simulink model "VtP_mod_3Bit"  (Simulink 7.9)
settings: Solver=ode45  StartTime=0.0  StopTime=simu.trantime  RelTol=1e-3
undefined symbols (not defined in the file): dc, Fs, mod, OSR, sinamp, sinfreq
libraries: dspsigattribs x14, dspsigops x9, dspmtrx3 x7, commblksprivate x7, commsrccod2 x7, dsparch4 x1, simulink x1, dspsrcs4 x1
settings Model: Creator=Isacco Arnaldi  LastModifiedBy=Arnaldi Isacco
settings SolverCC: ZcThreshold=1e-3  ZeroCrossAlgorithm=Adaptive  AutoInsertRateTranBlk=on
settings DataIOCC: LimitDataPoints=off  MaxDataPoints=50000  SaveOutput=off  SignalLogging=off  DSMLogging=off  SaveTime=off
settings OptimizationCC: InlineParams=on
settings DebuggingCC: SaveWithDisabledLinksMsg=none  SaveWithParameterizedLinksMsg=none  StrictBusMsg=Warning
settings ModelReferenceCC: ModelReferenceNumInstancesAllowed=Single
settings CodeAppCC: CustomSymbolStrType=$N$R$M_T
settings GRTTargetCC: CombineOutputUpdateFcns=off  GRTInterface=on
settings ConfigurationSet: Description=SimMechanics 2G

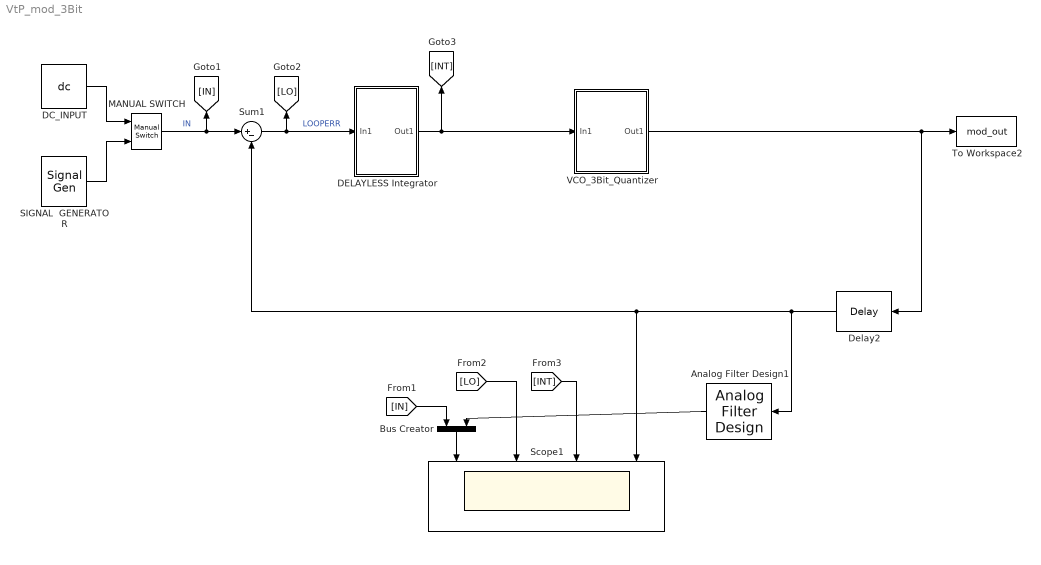
== system VtP_mod_3Bit ==
  Analog Filter Design1 : dsparch4/Analog Filter Design  method=Butterworth  filttype=Lowpass  N=8  Wlo=pi*(Fs/OSR)  Whi=80  Rp=2  Rs=40
  Bus Creator : BusCreator  Inputs=2
  DC_INPUT : Constant  Value=dc  VectorParams1D=off  OutDataTypeStr=double  SampleTime=1/Fs
  DELAYLESS Integrator : Subsystem
  Delay2 : dspsigops/Delay  InputProcessing=Inherited (this choice will be removed - see release notes)  dly_unit=Samples  delay=1  ic_detail=off  dif_ic_for_ch=off  dif_ic_for_dly=off  ic=0  reset_popup=None
  MANUAL SWITCH : simulink/Signal Routing/Manual Switch  sw=0  action=0  varsize=off
      settings: AttributesFormatString=Double click to\nselect the desired\ninput
  SIGNAL  GENERATOR : SignalGenerator  Amplitude=sinamp  Frequency=sinfreq  VectorParams1D=off
  Scope1 : Scope  NumInputPorts=4
      settings: TimeRange=2.089895171320487e-05  YMin=-1.1~-0.6~-0.6~-0.3  YMax=1.1~1.6~1.6~0.1
  Sum1 : Sum  Inputs=|+-  SampleTime=1/Fs
  To Workspace2 : ToWorkspace  VariableName=mod_out  SampleTime=-1
  VCO_3Bit_Quantizer : Subsystem
  wires:
  Sum1/1 -> [LO], DELAYLESS Integrator/1(In1)  "LOOPERR"
  DELAYLESS Integrator/1(Out1) -> [INT], VCO_3Bit_Quantizer/1(In1)
  Delay2/1 -> Analog Filter Design1/1, Sum1/2, Scope1/4
  DC_INPUT/1 -> MANUAL SWITCH/1
  SIGNAL  GENERATOR/1 -> MANUAL SWITCH/2
  MANUAL SWITCH/1 -> Sum1/1, [IN]  "IN"
  [IN] -> Bus Creator/1
  Bus Creator/1 -> Scope1/1
  Analog Filter Design1/1 -> Bus Creator/2
  [LO] -> Scope1/2
  [INT] -> Scope1/3
  VCO_3Bit_Quantizer/1(Out1) -> Delay2/1, To Workspace2/1

== system VtP_mod_3Bit/DELAYLESS Integrator ==
  In1 : Inport
  Delay1 : dspsigops/Delay  InputProcessing=Inherited (this choice will be removed - see release notes)  dly_unit=Samples  delay=1  ic_detail=off  dif_ic_for_ch=off  dif_ic_for_dly=off  ic=0  reset_popup=None
  Integrator pole : Gain  Gain=1-1/mod.igain1
      settings: AttributesFormatString=(model finite dc gain)
  Integrator saturation : Saturate  UpperLimit=mod.isat1  LowerLimit=-(mod.isat1)
  Sum : Sum  Inputs=|++  SampleTime=1/Fs
      settings: AttributesFormatString=Integrator summer
  Out1 : Outport
  wires:
  Integrator saturation/1 -> Integrator pole/1, Out1/1  "INT1OUT"
  In1/1 -> Sum/1
  Integrator pole/1 -> Delay1/1
  Delay1/1 -> Sum/2
  Sum/1 -> Integrator saturation/1  "INT1SUM"

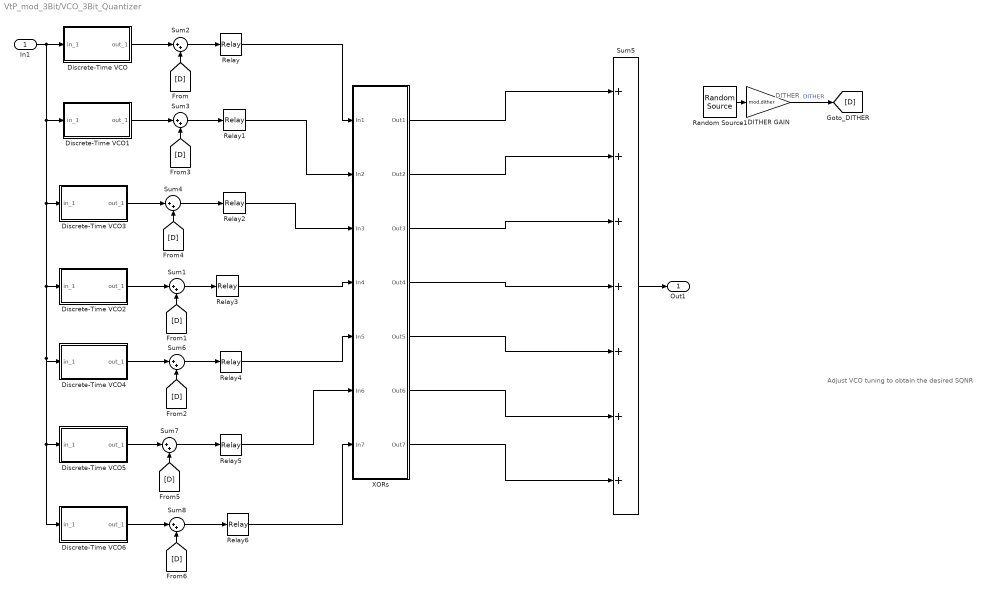
== system VtP_mod_3Bit/VCO_3Bit_Quantizer ==
  note: DITHER
  note: Adjust VCO tuning to obtain the desired SQNR
  In1 : Inport
  DITHER GAIN : Gain  Gain=mod.dither  SampleTime=1/Fs
  Discrete-Time VCO : Subsystem  AncestorBlock=commsynccomp2/Discrete-Time VCO  mask(Discrete-Time VCO){Ac=sinamp*2, Fc=Fs/100, Kc=sinfreq*5, Ph=0, ts=1/Fs}
      mask prompts: Ac "Output amplitude (V):"; Fc "Quiescent frequency (Hz):"; Kc "Input sensitivity (Hz/V):"; Ph "Initial phase (rad):"; ts "Sample time (s):"
      mask help: Generate a discrete-time output signal whose frequency changes in response to the amplitude variations of the input signal. The input signal must be a scalar.
      mask init:
      | if ( (length(Ac)~=1) || (length(Fc)~=1) || (length(Kc)~=1) || (length(Ph)~=1) || (length(ts)~=1) ) 
      | 	error('commblks:DiscTimeVCO:InvalidMaskParams',...
      |           'Mask parameters must be scalar values.');
      | end
      | FcRadians = 2*pi*Fc;
      | KcRadPerV = 2*pi*Kc;
      mask Help: helpview(commbhelp)
      mask Display: disp('Discrete-Time\nVCO')
  Discrete-Time VCO1 : Subsystem  AncestorBlock=commsynccomp2/Discrete-Time VCO  mask(Discrete-Time VCO){Ac=sinamp*2, Fc=Fs/100, Kc=sinfreq*5, Ph=0.4487, ts=1/Fs}
      mask prompts: Ac "Output amplitude (V):"; Fc "Quiescent frequency (Hz):"; Kc "Input sensitivity (Hz/V):"; Ph "Initial phase (rad):"; ts "Sample time (s):"
      mask help: Generate a discrete-time output signal whose frequency changes in response to the amplitude variations of the input signal. The input signal must be a scalar.
      mask init: same as VtP_mod_3Bit/VCO_3Bit_Quantizer/Discrete-Time VCO
      mask Help: helpview(commbhelp)
      mask Display: disp('Discrete-Time\nVCO')
  Discrete-Time VCO2 : Subsystem  AncestorBlock=commsynccomp2/Discrete-Time VCO  mask(Discrete-Time VCO){Ac=sinamp*2, Fc=Fs/100, Kc=sinfreq*5, Ph=1.34, ts=1/Fs}
      mask prompts: Ac "Output amplitude (V):"; Fc "Quiescent frequency (Hz):"; Kc "Input sensitivity (Hz/V):"; Ph "Initial phase (rad):"; ts "Sample time (s):"
      mask help: Generate a discrete-time output signal whose frequency changes in response to the amplitude variations of the input signal. The input signal must be a scalar.
      mask init: same as VtP_mod_3Bit/VCO_3Bit_Quantizer/Discrete-Time VCO
      mask Help: helpview(commbhelp)
      mask Display: disp('Discrete-Time\nVCO')
  Discrete-Time VCO3 : Subsystem  AncestorBlock=commsynccomp2/Discrete-Time VCO  mask(Discrete-Time VCO){Ac=sinamp*2, Fc=Fs/10, Kc=sinfreq*5, Ph=0.89, ts=1/Fs}
      mask prompts: Ac "Output amplitude (V):"; Fc "Quiescent frequency (Hz):"; Kc "Input sensitivity (Hz/V):"; Ph "Initial phase (rad):"; ts "Sample time (s):"
      mask help: Generate a discrete-time output signal whose frequency changes in response to the amplitude variations of the input signal. The input signal must be a scalar.
      mask init: same as VtP_mod_3Bit/VCO_3Bit_Quantizer/Discrete-Time VCO
      mask Help: helpview(commbhelp)
      mask Display: disp('Discrete-Time\nVCO')
  Discrete-Time VCO4 : Subsystem  AncestorBlock=commsynccomp2/Discrete-Time VCO  mask(Discrete-Time VCO){Ac=sinamp*2, Fc=Fs/100, Kc=sinfreq*5, Ph=1.79, ts=1/Fs}
      mask prompts: Ac "Output amplitude (V):"; Fc "Quiescent frequency (Hz):"; Kc "Input sensitivity (Hz/V):"; Ph "Initial phase (rad):"; ts "Sample time (s):"
      mask help: Generate a discrete-time output signal whose frequency changes in response to the amplitude variations of the input signal. The input signal must be a scalar.
      mask init: same as VtP_mod_3Bit/VCO_3Bit_Quantizer/Discrete-Time VCO
      mask Help: helpview(commbhelp)
      mask Display: disp('Discrete-Time\nVCO')
  Discrete-Time VCO5 : Subsystem  AncestorBlock=commsynccomp2/Discrete-Time VCO  mask(Discrete-Time VCO){Ac=sinamp*2, Fc=Fs/100, Kc=sinfreq*5, Ph=2.24, ts=1/Fs}
      mask prompts: Ac "Output amplitude (V):"; Fc "Quiescent frequency (Hz):"; Kc "Input sensitivity (Hz/V):"; Ph "Initial phase (rad):"; ts "Sample time (s):"
      mask help: Generate a discrete-time output signal whose frequency changes in response to the amplitude variations of the input signal. The input signal must be a scalar.
      mask init: same as VtP_mod_3Bit/VCO_3Bit_Quantizer/Discrete-Time VCO
      mask Help: helpview(commbhelp)
      mask Display: disp('Discrete-Time\nVCO')
  Discrete-Time VCO6 : Subsystem  AncestorBlock=commsynccomp2/Discrete-Time VCO  mask(Discrete-Time VCO){Ac=sinamp*2, Fc=Fs/100, Kc=sinfreq*5, Ph=3.14, ts=1/Fs}
      mask prompts: Ac "Output amplitude (V):"; Fc "Quiescent frequency (Hz):"; Kc "Input sensitivity (Hz/V):"; Ph "Initial phase (rad):"; ts "Sample time (s):"
      mask help: Generate a discrete-time output signal whose frequency changes in response to the amplitude variations of the input signal. The input signal must be a scalar.
      mask init: same as VtP_mod_3Bit/VCO_3Bit_Quantizer/Discrete-Time VCO
      mask Help: helpview(commbhelp)
      mask Display: disp('Discrete-Time\nVCO')
  Random Source1 : dspsrcs4/Random Source  SrcType=Uniform  NormMethod=Ziggurat  CltLength=12  MinVal=-1  MaxVal=1  MeanVal=0  VarVal=1  RepMode=Not repeatable  rawSeed=1  IsInherit=off  SampMode=Discrete  SampTime=1/Fs  SampFrame=1  DataType=Double  OutComplex=Real
  Relay{,1..6} (7 alike) : Relay  SampleTime=1/Fs
  Sum{1..4,6..8} (7 alike) : Sum  Inputs=|++  SampleTime=1/Fs
  Sum5 : Sum  Inputs=+++++++  SampleTime=1/Fs
  XORs : Subsystem
  Out1 : Outport
  wires:
  [D] -> Sum2/2
  Discrete-Time VCO/1(out_1) -> Sum2/1
  [D] -> Sum3/2
  Discrete-Time VCO1/1(out_1) -> Sum3/1
  [D] -> Sum4/2
  Sum4/1 -> Relay2/1
  Discrete-Time VCO3/1(out_1) -> Sum4/1
  Sum2/1 -> Relay/1
  Relay/1 -> XORs/1(In1)
  Sum3/1 -> Relay1/1
  Relay1/1 -> XORs/2(In2)
  In1/1 -> Discrete-Time VCO/1(in_1), Discrete-Time VCO1/1(in_1), Discrete-Time VCO3/1(in_1), Discrete-Time VCO2/1(in_1), Discrete-Time VCO4/1(in_1), Discrete-Time VCO5/1(in_1), Discrete-Time VCO6/1(in_1)
  [D] -> Sum1/2
  Discrete-Time VCO2/1(out_1) -> Sum1/1
  [D] -> Sum6/2
  Discrete-Time VCO4/1(out_1) -> Sum6/1
  [D] -> Sum7/2
  Sum7/1 -> Relay5/1
  Discrete-Time VCO5/1(out_1) -> Sum7/1
  Sum1/1 -> Relay3/1
  Relay3/1 -> XORs/4(In4)
  Sum6/1 -> Relay4/1
  Relay4/1 -> XORs/5(In5)
  Relay5/1 -> XORs/6(In6)
  [D] -> Sum8/2
  Sum8/1 -> Relay6/1
  Discrete-Time VCO6/1(out_1) -> Sum8/1
  Relay6/1 -> XORs/7(In7)
  Random Source1/1 -> DITHER GAIN/1
  DITHER GAIN/1 -> [D]  "DITHER"
  Sum5/1 -> Out1/1
  Relay2/1 -> XORs/3(In3)
  XORs/7(Out7) -> Sum5/7
  XORs/6(Out6) -> Sum5/6
  XORs/5(Out5) -> Sum5/5
  XORs/4(Out4) -> Sum5/4
  XORs/3(Out3) -> Sum5/3
  XORs/2(Out2) -> Sum5/2
  XORs/1(Out1) -> Sum5/1

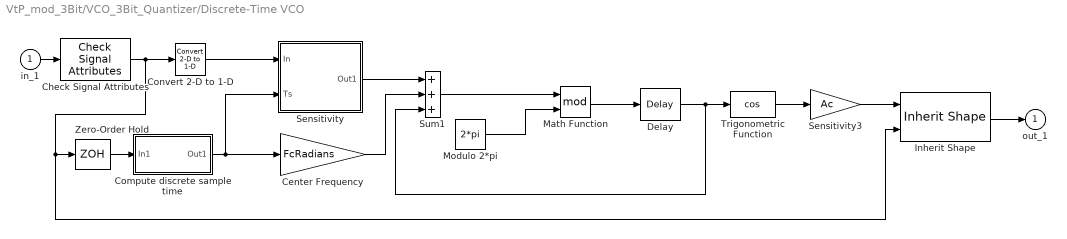
== system VtP_mod_3Bit/VCO_3Bit_Quantizer/Discrete-Time VCO ==
  in_1 : Inport
  Center Frequency : Gain  Gain=FcRadians  ParamDataTypeStr=float('double')  OutDataTypeStr=Inherit: Inherit via back propagation  RndMeth=Nearest  SampleTime=ts  SaturateOnIntegerOverflow=on
  Check Signal Attributes : dspsigattribs/Check Signal Attributes  SigAttribCheckMethod=Does not match attributes exactly  Complexity=Ignore  Frame=Ignore  DimsCheckMethod=Is...  Dimensions=Scalar (1-D or 2-D)  DatatypeCheckMethod=Is...  DatatypeGeneral=Floating-point  DtypeFloatSpecific=Any floating-point  DtypeFixedSpecific=Any fixed-point  DtypeIntSpecific=Any integer  SampleMode=Discrete
  Compute discrete sample time : Subsystem
  Convert 2-D to 1-D : dspsigattribs/Convert 2-D to 1-D
  Delay : dspsigops/Delay  InputProcessing=Columns as channels (frame based)  dly_unit=Samples  delay=1  ic_detail=on  dif_ic_for_ch=off  dif_ic_for_dly=off  ic=Ph  reset_popup=None
  Inherit Shape : commblksprivate/Inherit Shape
  Math Function : Math  Operator=mod  SaturateOnIntegerOverflow=on
  Modulo 2*pi : Constant  Value=2*pi  OutDataTypeStr=Inherit: Inherit via back propagation  SampleTime=ts
  Sensitivity : Subsystem
  Sensitivity3 : Gain  Gain=Ac  SaturateOnIntegerOverflow=on  OutDataTypeStr=Inherit: Same as input  ParamDataTypeStr=Inherit: Same as input
  Sum1 : Sum  Inputs=+++  SaturateOnIntegerOverflow=on  InputSameDT=on  OutDataTypeStr=Inherit: Same as first input
  Trigonometric Function : Trigonometry  Operator=cos
  Zero-Order Hold : ZeroOrderHold  SampleTime=ts
  out_1 : Outport  InitialOutput=0
  wires:
  Zero-Order Hold/1 -> Compute discrete sample time/1(In1)
  Sensitivity/1(Out1) -> Sum1/1
  Compute discrete sample time/1(Out1) -> Sensitivity/2(Ts), Center Frequency/1
  Center Frequency/1 -> Sum1/2
  Check Signal Attributes/1 -> Inherit Shape/2, Zero-Order Hold/1, Convert 2-D to 1-D/1
  Trigonometric Function/1 -> Sensitivity3/1
  in_1/1 -> Check Signal Attributes/1
  Math Function/1 -> Delay/1
  Sum1/1 -> Math Function/1
  Modulo 2*pi/1 -> Math Function/2
  Convert 2-D to 1-D/1 -> Sensitivity/1(In)
  Sensitivity3/1 -> Inherit Shape/1
  Inherit Shape/1 -> out_1/1
  Delay/1 -> Trigonometric Function/1, Sum1/3

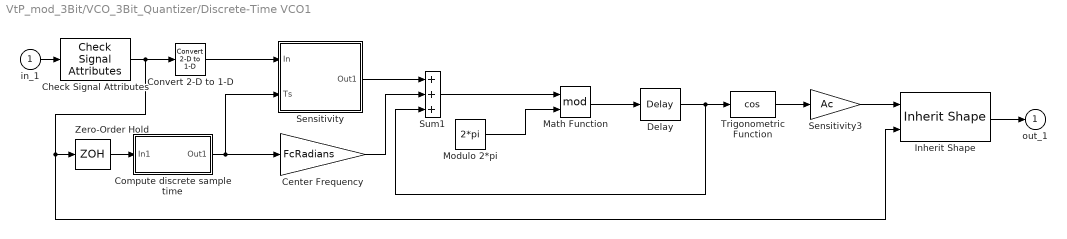
== system VtP_mod_3Bit/VCO_3Bit_Quantizer/Discrete-Time VCO1 ==
  in_1 : Inport
  Center Frequency : Gain  Gain=FcRadians  ParamDataTypeStr=float('double')  OutDataTypeStr=Inherit: Inherit via back propagation  RndMeth=Nearest  SampleTime=ts  SaturateOnIntegerOverflow=on
  Check Signal Attributes : dspsigattribs/Check Signal Attributes  SigAttribCheckMethod=Does not match attributes exactly  Complexity=Ignore  Frame=Ignore  DimsCheckMethod=Is...  Dimensions=Scalar (1-D or 2-D)  DatatypeCheckMethod=Is...  DatatypeGeneral=Floating-point  DtypeFloatSpecific=Any floating-point  DtypeFixedSpecific=Any fixed-point  DtypeIntSpecific=Any integer  SampleMode=Discrete
  Compute discrete sample time : Subsystem
  Convert 2-D to 1-D : dspsigattribs/Convert 2-D to 1-D
  Delay : dspsigops/Delay  InputProcessing=Columns as channels (frame based)  dly_unit=Samples  delay=1  ic_detail=on  dif_ic_for_ch=off  dif_ic_for_dly=off  ic=Ph  reset_popup=None
  Inherit Shape : commblksprivate/Inherit Shape
  Math Function : Math  Operator=mod  SaturateOnIntegerOverflow=on
  Modulo 2*pi : Constant  Value=2*pi  OutDataTypeStr=Inherit: Inherit via back propagation  SampleTime=ts
  Sensitivity : Subsystem
  Sensitivity3 : Gain  Gain=Ac  SaturateOnIntegerOverflow=on  OutDataTypeStr=Inherit: Same as input  ParamDataTypeStr=Inherit: Same as input
  Sum1 : Sum  Inputs=+++  SaturateOnIntegerOverflow=on  InputSameDT=on  OutDataTypeStr=Inherit: Same as first input
  Trigonometric Function : Trigonometry  Operator=cos
  Zero-Order Hold : ZeroOrderHold  SampleTime=ts
  out_1 : Outport  InitialOutput=0
  wires:
  Zero-Order Hold/1 -> Compute discrete sample time/1(In1)
  Sensitivity/1(Out1) -> Sum1/1
  Compute discrete sample time/1(Out1) -> Sensitivity/2(Ts), Center Frequency/1
  Center Frequency/1 -> Sum1/2
  Check Signal Attributes/1 -> Inherit Shape/2, Zero-Order Hold/1, Convert 2-D to 1-D/1
  Trigonometric Function/1 -> Sensitivity3/1
  in_1/1 -> Check Signal Attributes/1
  Math Function/1 -> Delay/1
  Sum1/1 -> Math Function/1
  Modulo 2*pi/1 -> Math Function/2
  Convert 2-D to 1-D/1 -> Sensitivity/1(In)
  Sensitivity3/1 -> Inherit Shape/1
  Inherit Shape/1 -> out_1/1
  Delay/1 -> Trigonometric Function/1, Sum1/3

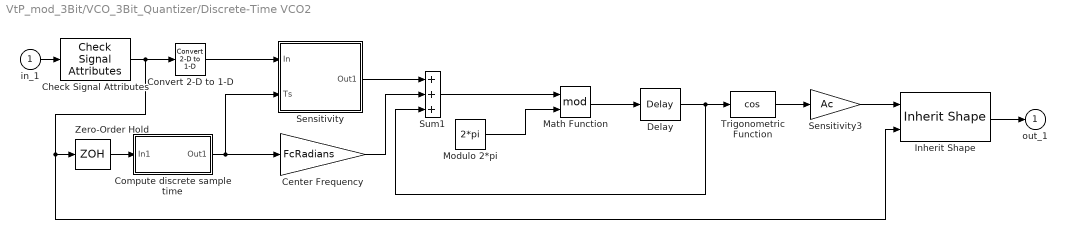
== system VtP_mod_3Bit/VCO_3Bit_Quantizer/Discrete-Time VCO2 ==
  in_1 : Inport
  Center Frequency : Gain  Gain=FcRadians  ParamDataTypeStr=float('double')  OutDataTypeStr=Inherit: Inherit via back propagation  RndMeth=Nearest  SampleTime=ts  SaturateOnIntegerOverflow=on
  Check Signal Attributes : dspsigattribs/Check Signal Attributes  SigAttribCheckMethod=Does not match attributes exactly  Complexity=Ignore  Frame=Ignore  DimsCheckMethod=Is...  Dimensions=Scalar (1-D or 2-D)  DatatypeCheckMethod=Is...  DatatypeGeneral=Floating-point  DtypeFloatSpecific=Any floating-point  DtypeFixedSpecific=Any fixed-point  DtypeIntSpecific=Any integer  SampleMode=Discrete
  Compute discrete sample time : Subsystem
  Convert 2-D to 1-D : dspsigattribs/Convert 2-D to 1-D
  Delay : dspsigops/Delay  InputProcessing=Columns as channels (frame based)  dly_unit=Samples  delay=1  ic_detail=on  dif_ic_for_ch=off  dif_ic_for_dly=off  ic=Ph  reset_popup=None
  Inherit Shape : commblksprivate/Inherit Shape
  Math Function : Math  Operator=mod  SaturateOnIntegerOverflow=on
  Modulo 2*pi : Constant  Value=2*pi  OutDataTypeStr=Inherit: Inherit via back propagation  SampleTime=ts
  Sensitivity : Subsystem
  Sensitivity3 : Gain  Gain=Ac  SaturateOnIntegerOverflow=on  OutDataTypeStr=Inherit: Same as input  ParamDataTypeStr=Inherit: Same as input
  Sum1 : Sum  Inputs=+++  SaturateOnIntegerOverflow=on  InputSameDT=on  OutDataTypeStr=Inherit: Same as first input
  Trigonometric Function : Trigonometry  Operator=cos
  Zero-Order Hold : ZeroOrderHold  SampleTime=ts
  out_1 : Outport  InitialOutput=0
  wires:
  Zero-Order Hold/1 -> Compute discrete sample time/1(In1)
  Sensitivity/1(Out1) -> Sum1/1
  Compute discrete sample time/1(Out1) -> Sensitivity/2(Ts), Center Frequency/1
  Center Frequency/1 -> Sum1/2
  Check Signal Attributes/1 -> Inherit Shape/2, Zero-Order Hold/1, Convert 2-D to 1-D/1
  Trigonometric Function/1 -> Sensitivity3/1
  in_1/1 -> Check Signal Attributes/1
  Math Function/1 -> Delay/1
  Sum1/1 -> Math Function/1
  Modulo 2*pi/1 -> Math Function/2
  Convert 2-D to 1-D/1 -> Sensitivity/1(In)
  Sensitivity3/1 -> Inherit Shape/1
  Inherit Shape/1 -> out_1/1
  Delay/1 -> Trigonometric Function/1, Sum1/3

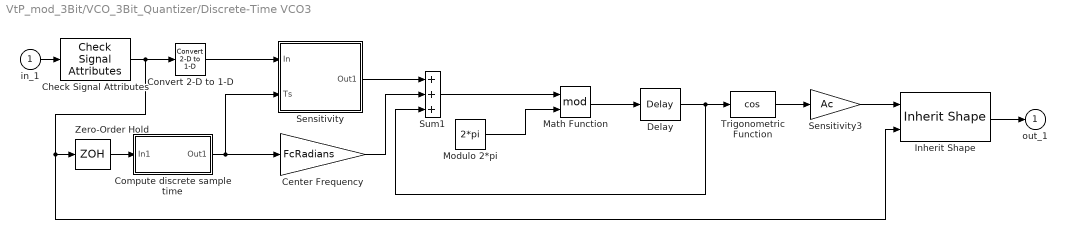
== system VtP_mod_3Bit/VCO_3Bit_Quantizer/Discrete-Time VCO3 ==
  in_1 : Inport
  Center Frequency : Gain  Gain=FcRadians  ParamDataTypeStr=float('double')  OutDataTypeStr=Inherit: Inherit via back propagation  RndMeth=Nearest  SampleTime=ts  SaturateOnIntegerOverflow=on
  Check Signal Attributes : dspsigattribs/Check Signal Attributes  SigAttribCheckMethod=Does not match attributes exactly  Complexity=Ignore  Frame=Ignore  DimsCheckMethod=Is...  Dimensions=Scalar (1-D or 2-D)  DatatypeCheckMethod=Is...  DatatypeGeneral=Floating-point  DtypeFloatSpecific=Any floating-point  DtypeFixedSpecific=Any fixed-point  DtypeIntSpecific=Any integer  SampleMode=Discrete
  Compute discrete sample time : Subsystem
  Convert 2-D to 1-D : dspsigattribs/Convert 2-D to 1-D
  Delay : dspsigops/Delay  InputProcessing=Columns as channels (frame based)  dly_unit=Samples  delay=1  ic_detail=on  dif_ic_for_ch=off  dif_ic_for_dly=off  ic=Ph  reset_popup=None
  Inherit Shape : commblksprivate/Inherit Shape
  Math Function : Math  Operator=mod  SaturateOnIntegerOverflow=on
  Modulo 2*pi : Constant  Value=2*pi  OutDataTypeStr=Inherit: Inherit via back propagation  SampleTime=ts
  Sensitivity : Subsystem
  Sensitivity3 : Gain  Gain=Ac  SaturateOnIntegerOverflow=on  OutDataTypeStr=Inherit: Same as input  ParamDataTypeStr=Inherit: Same as input
  Sum1 : Sum  Inputs=+++  SaturateOnIntegerOverflow=on  InputSameDT=on  OutDataTypeStr=Inherit: Same as first input
  Trigonometric Function : Trigonometry  Operator=cos
  Zero-Order Hold : ZeroOrderHold  SampleTime=ts
  out_1 : Outport  InitialOutput=0
  wires:
  Zero-Order Hold/1 -> Compute discrete sample time/1(In1)
  Sensitivity/1(Out1) -> Sum1/1
  Compute discrete sample time/1(Out1) -> Sensitivity/2(Ts), Center Frequency/1
  Center Frequency/1 -> Sum1/2
  Check Signal Attributes/1 -> Inherit Shape/2, Zero-Order Hold/1, Convert 2-D to 1-D/1
  Trigonometric Function/1 -> Sensitivity3/1
  in_1/1 -> Check Signal Attributes/1
  Math Function/1 -> Delay/1
  Sum1/1 -> Math Function/1
  Modulo 2*pi/1 -> Math Function/2
  Convert 2-D to 1-D/1 -> Sensitivity/1(In)
  Sensitivity3/1 -> Inherit Shape/1
  Inherit Shape/1 -> out_1/1
  Delay/1 -> Trigonometric Function/1, Sum1/3

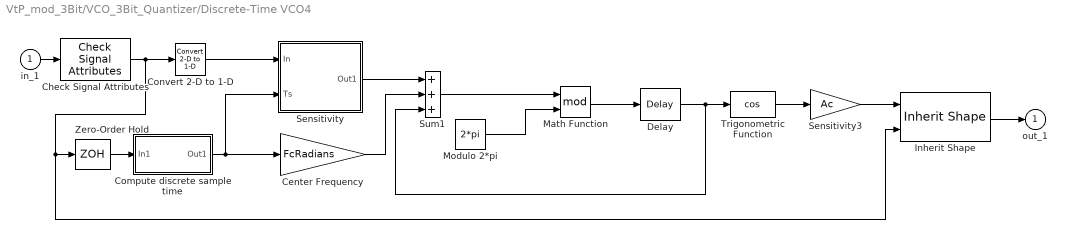
== system VtP_mod_3Bit/VCO_3Bit_Quantizer/Discrete-Time VCO4 ==
  in_1 : Inport
  Center Frequency : Gain  Gain=FcRadians  ParamDataTypeStr=float('double')  OutDataTypeStr=Inherit: Inherit via back propagation  RndMeth=Nearest  SampleTime=ts  SaturateOnIntegerOverflow=on
  Check Signal Attributes : dspsigattribs/Check Signal Attributes  SigAttribCheckMethod=Does not match attributes exactly  Complexity=Ignore  Frame=Ignore  DimsCheckMethod=Is...  Dimensions=Scalar (1-D or 2-D)  DatatypeCheckMethod=Is...  DatatypeGeneral=Floating-point  DtypeFloatSpecific=Any floating-point  DtypeFixedSpecific=Any fixed-point  DtypeIntSpecific=Any integer  SampleMode=Discrete
  Compute discrete sample time : Subsystem
  Convert 2-D to 1-D : dspsigattribs/Convert 2-D to 1-D
  Delay : dspsigops/Delay  InputProcessing=Columns as channels (frame based)  dly_unit=Samples  delay=1  ic_detail=on  dif_ic_for_ch=off  dif_ic_for_dly=off  ic=Ph  reset_popup=None
  Inherit Shape : commblksprivate/Inherit Shape
  Math Function : Math  Operator=mod  SaturateOnIntegerOverflow=on
  Modulo 2*pi : Constant  Value=2*pi  OutDataTypeStr=Inherit: Inherit via back propagation  SampleTime=ts
  Sensitivity : Subsystem
  Sensitivity3 : Gain  Gain=Ac  SaturateOnIntegerOverflow=on  OutDataTypeStr=Inherit: Same as input  ParamDataTypeStr=Inherit: Same as input
  Sum1 : Sum  Inputs=+++  SaturateOnIntegerOverflow=on  InputSameDT=on  OutDataTypeStr=Inherit: Same as first input
  Trigonometric Function : Trigonometry  Operator=cos
  Zero-Order Hold : ZeroOrderHold  SampleTime=ts
  out_1 : Outport  InitialOutput=0
  wires:
  Zero-Order Hold/1 -> Compute discrete sample time/1(In1)
  Sensitivity/1(Out1) -> Sum1/1
  Compute discrete sample time/1(Out1) -> Sensitivity/2(Ts), Center Frequency/1
  Center Frequency/1 -> Sum1/2
  Check Signal Attributes/1 -> Inherit Shape/2, Zero-Order Hold/1, Convert 2-D to 1-D/1
  Trigonometric Function/1 -> Sensitivity3/1
  in_1/1 -> Check Signal Attributes/1
  Math Function/1 -> Delay/1
  Sum1/1 -> Math Function/1
  Modulo 2*pi/1 -> Math Function/2
  Convert 2-D to 1-D/1 -> Sensitivity/1(In)
  Sensitivity3/1 -> Inherit Shape/1
  Inherit Shape/1 -> out_1/1
  Delay/1 -> Trigonometric Function/1, Sum1/3

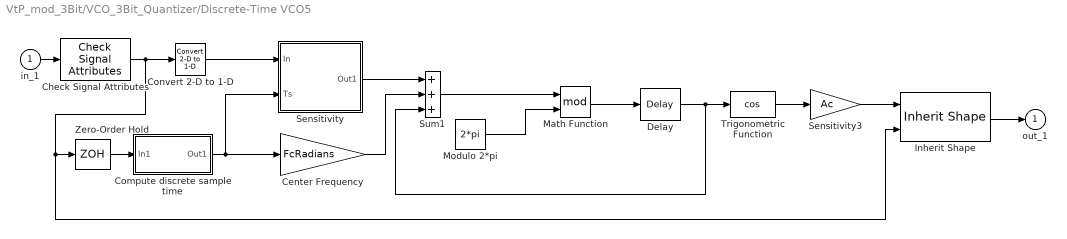
== system VtP_mod_3Bit/VCO_3Bit_Quantizer/Discrete-Time VCO5 ==
  in_1 : Inport
  Center Frequency : Gain  Gain=FcRadians  ParamDataTypeStr=float('double')  OutDataTypeStr=Inherit: Inherit via back propagation  RndMeth=Nearest  SampleTime=ts  SaturateOnIntegerOverflow=on
  Check Signal Attributes : dspsigattribs/Check Signal Attributes  SigAttribCheckMethod=Does not match attributes exactly  Complexity=Ignore  Frame=Ignore  DimsCheckMethod=Is...  Dimensions=Scalar (1-D or 2-D)  DatatypeCheckMethod=Is...  DatatypeGeneral=Floating-point  DtypeFloatSpecific=Any floating-point  DtypeFixedSpecific=Any fixed-point  DtypeIntSpecific=Any integer  SampleMode=Discrete
  Compute discrete sample time : Subsystem
  Convert 2-D to 1-D : dspsigattribs/Convert 2-D to 1-D
  Delay : dspsigops/Delay  InputProcessing=Columns as channels (frame based)  dly_unit=Samples  delay=1  ic_detail=on  dif_ic_for_ch=off  dif_ic_for_dly=off  ic=Ph  reset_popup=None
  Inherit Shape : commblksprivate/Inherit Shape
  Math Function : Math  Operator=mod  SaturateOnIntegerOverflow=on
  Modulo 2*pi : Constant  Value=2*pi  OutDataTypeStr=Inherit: Inherit via back propagation  SampleTime=ts
  Sensitivity : Subsystem
  Sensitivity3 : Gain  Gain=Ac  SaturateOnIntegerOverflow=on  OutDataTypeStr=Inherit: Same as input  ParamDataTypeStr=Inherit: Same as input
  Sum1 : Sum  Inputs=+++  SaturateOnIntegerOverflow=on  InputSameDT=on  OutDataTypeStr=Inherit: Same as first input
  Trigonometric Function : Trigonometry  Operator=cos
  Zero-Order Hold : ZeroOrderHold  SampleTime=ts
  out_1 : Outport  InitialOutput=0
  wires:
  Zero-Order Hold/1 -> Compute discrete sample time/1(In1)
  Sensitivity/1(Out1) -> Sum1/1
  Compute discrete sample time/1(Out1) -> Sensitivity/2(Ts), Center Frequency/1
  Center Frequency/1 -> Sum1/2
  Check Signal Attributes/1 -> Inherit Shape/2, Zero-Order Hold/1, Convert 2-D to 1-D/1
  Trigonometric Function/1 -> Sensitivity3/1
  in_1/1 -> Check Signal Attributes/1
  Math Function/1 -> Delay/1
  Sum1/1 -> Math Function/1
  Modulo 2*pi/1 -> Math Function/2
  Convert 2-D to 1-D/1 -> Sensitivity/1(In)
  Sensitivity3/1 -> Inherit Shape/1
  Inherit Shape/1 -> out_1/1
  Delay/1 -> Trigonometric Function/1, Sum1/3

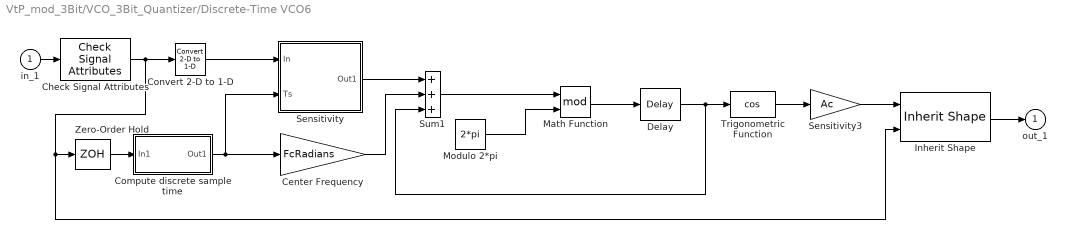
== system VtP_mod_3Bit/VCO_3Bit_Quantizer/Discrete-Time VCO6 ==
  in_1 : Inport
  Center Frequency : Gain  Gain=FcRadians  ParamDataTypeStr=float('double')  OutDataTypeStr=Inherit: Inherit via back propagation  RndMeth=Nearest  SampleTime=ts  SaturateOnIntegerOverflow=on
  Check Signal Attributes : dspsigattribs/Check Signal Attributes  SigAttribCheckMethod=Does not match attributes exactly  Complexity=Ignore  Frame=Ignore  DimsCheckMethod=Is...  Dimensions=Scalar (1-D or 2-D)  DatatypeCheckMethod=Is...  DatatypeGeneral=Floating-point  DtypeFloatSpecific=Any floating-point  DtypeFixedSpecific=Any fixed-point  DtypeIntSpecific=Any integer  SampleMode=Discrete
  Compute discrete sample time : Subsystem
  Convert 2-D to 1-D : dspsigattribs/Convert 2-D to 1-D
  Delay : dspsigops/Delay  InputProcessing=Columns as channels (frame based)  dly_unit=Samples  delay=1  ic_detail=on  dif_ic_for_ch=off  dif_ic_for_dly=off  ic=Ph  reset_popup=None
  Inherit Shape : commblksprivate/Inherit Shape
  Math Function : Math  Operator=mod  SaturateOnIntegerOverflow=on
  Modulo 2*pi : Constant  Value=2*pi  OutDataTypeStr=Inherit: Inherit via back propagation  SampleTime=ts
  Sensitivity : Subsystem
  Sensitivity3 : Gain  Gain=Ac  SaturateOnIntegerOverflow=on  OutDataTypeStr=Inherit: Same as input  ParamDataTypeStr=Inherit: Same as input
  Sum1 : Sum  Inputs=+++  SaturateOnIntegerOverflow=on  InputSameDT=on  OutDataTypeStr=Inherit: Same as first input
  Trigonometric Function : Trigonometry  Operator=cos
  Zero-Order Hold : ZeroOrderHold  SampleTime=ts
  out_1 : Outport  InitialOutput=0
  wires:
  Zero-Order Hold/1 -> Compute discrete sample time/1(In1)
  Sensitivity/1(Out1) -> Sum1/1
  Compute discrete sample time/1(Out1) -> Sensitivity/2(Ts), Center Frequency/1
  Center Frequency/1 -> Sum1/2
  Check Signal Attributes/1 -> Inherit Shape/2, Zero-Order Hold/1, Convert 2-D to 1-D/1
  Trigonometric Function/1 -> Sensitivity3/1
  in_1/1 -> Check Signal Attributes/1
  Math Function/1 -> Delay/1
  Sum1/1 -> Math Function/1
  Modulo 2*pi/1 -> Math Function/2
  Convert 2-D to 1-D/1 -> Sensitivity/1(In)
  Sensitivity3/1 -> Inherit Shape/1
  Inherit Shape/1 -> out_1/1
  Delay/1 -> Trigonometric Function/1, Sum1/3

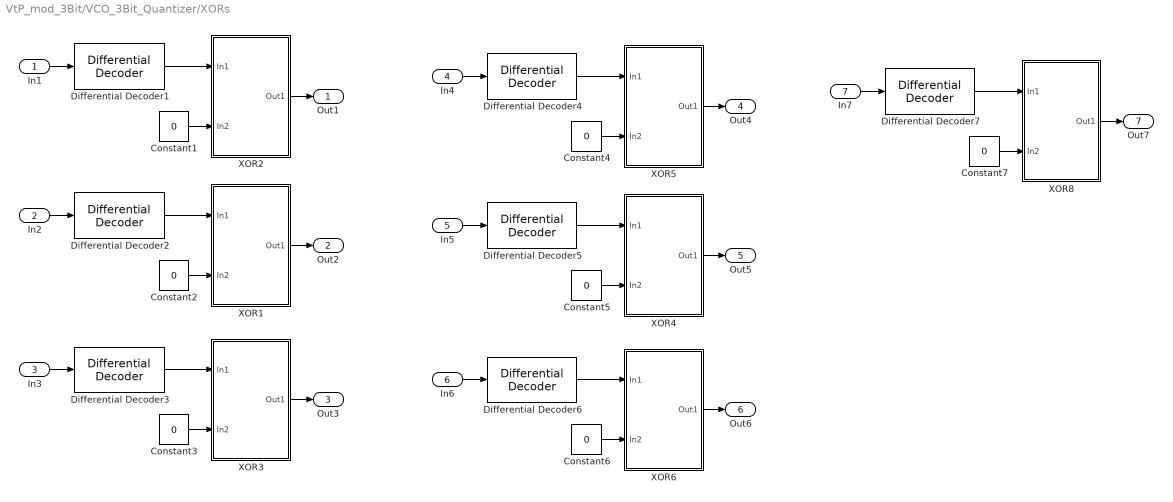
== system VtP_mod_3Bit/VCO_3Bit_Quantizer/XORs ==
  In1 : Inport
  In2 : Inport  Port=2
  In3 : Inport  Port=3
  In4 : Inport  Port=4
  In5 : Inport  Port=5
  In6 : Inport  Port=6
  In7 : Inport  Port=7
  Constant{1..7} (7 alike) : Constant  Value=0  VectorParams1D=off  OutDataTypeStr=boolean  SampleTime=1/Fs
  Differential Decoder{1..7} (7 alike) : commsrccod2/Differential Decoder  InitCond=0
  XOR1 : Subsystem
  XOR2 : Subsystem
  XOR3 : Subsystem
  XOR4 : Subsystem
  XOR5 : Subsystem
  XOR6 : Subsystem
  XOR8 : Subsystem
  Out1 : Outport
  Out2 : Outport  Port=2
  Out3 : Outport  Port=3
  Out4 : Outport  Port=4
  Out5 : Outport  Port=5
  Out6 : Outport  Port=6
  Out7 : Outport  Port=7
  wires:
  Constant1/1 -> XOR2/2(In2)
  Differential Decoder1/1 -> XOR2/1(In1)
  Constant2/1 -> XOR1/2(In2)
  Differential Decoder2/1 -> XOR1/1(In1)
  Constant3/1 -> XOR3/2(In2)
  Differential Decoder3/1 -> XOR3/1(In1)
  In1/1 -> Differential Decoder1/1
  XOR2/1(Out1) -> Out1/1
  In2/1 -> Differential Decoder2/1
  XOR1/1(Out1) -> Out2/1
  In3/1 -> Differential Decoder3/1
  XOR3/1(Out1) -> Out3/1
  Constant4/1 -> XOR5/2(In2)
  Differential Decoder4/1 -> XOR5/1(In1)
  Constant5/1 -> XOR4/2(In2)
  Differential Decoder5/1 -> XOR4/1(In1)
  Constant6/1 -> XOR6/2(In2)
  Differential Decoder6/1 -> XOR6/1(In1)
  In4/1 -> Differential Decoder4/1
  XOR5/1(Out1) -> Out4/1
  In5/1 -> Differential Decoder5/1
  XOR4/1(Out1) -> Out5/1
  In6/1 -> Differential Decoder6/1
  XOR6/1(Out1) -> Out6/1
  Constant7/1 -> XOR8/2(In2)
  Differential Decoder7/1 -> XOR8/1(In1)
  In7/1 -> Differential Decoder7/1
  XOR8/1(Out1) -> Out7/1

== system VtP_mod_3Bit/VCO_3Bit_Quantizer/Discrete-Time VCO/Compute discrete sample time ==
  In1 : Inport
  Probe : Probe  ProbeWidth=off  ProbeComplexSignal=off
  Submatrix : dspmtrx3/Submatrix  RowSpan=One row  RowStartMode=First  RowStartIndex=1  RowEndMode=Last  RowEndIndex=1  ColSpan=One column  ColStartMode=First  ColStartIndex=1  ColEndMode=Last  ColEndIndex=1
  Out1 : Outport
  wires:
  Submatrix/1 -> Out1/1
  In1/1 -> Probe/1
  Probe/1 -> Submatrix/1

== system VtP_mod_3Bit/VCO_3Bit_Quantizer/Discrete-Time VCO/Sensitivity ==
  In : Inport
  Ts : Inport  Port=2
  Gain : Gain  Gain=KcRadPerV  ParamDataTypeStr=float('double')  SaturateOnIntegerOverflow=on  OutDataTypeStr=Inherit: Same as input
  Product : Product  RndMeth=Nearest  SaturateOnIntegerOverflow=on  OutDataTypeStr=Inherit: Same as first input
  Out1 : Outport
  wires:
  Product/1 -> Out1/1
  In/1 -> Gain/1
  Ts/1 -> Product/2
  Gain/1 -> Product/1

== system VtP_mod_3Bit/VCO_3Bit_Quantizer/Discrete-Time VCO1/Compute discrete sample time ==
  In1 : Inport
  Probe : Probe  ProbeWidth=off  ProbeComplexSignal=off
  Submatrix : dspmtrx3/Submatrix  RowSpan=One row  RowStartMode=First  RowStartIndex=1  RowEndMode=Last  RowEndIndex=1  ColSpan=One column  ColStartMode=First  ColStartIndex=1  ColEndMode=Last  ColEndIndex=1
  Out1 : Outport
  wires:
  Submatrix/1 -> Out1/1
  In1/1 -> Probe/1
  Probe/1 -> Submatrix/1

== system VtP_mod_3Bit/VCO_3Bit_Quantizer/Discrete-Time VCO1/Sensitivity ==
  In : Inport
  Ts : Inport  Port=2
  Gain : Gain  Gain=KcRadPerV  ParamDataTypeStr=float('double')  SaturateOnIntegerOverflow=on  OutDataTypeStr=Inherit: Same as input
  Product : Product  RndMeth=Nearest  SaturateOnIntegerOverflow=on  OutDataTypeStr=Inherit: Same as first input
  Out1 : Outport
  wires:
  Product/1 -> Out1/1
  In/1 -> Gain/1
  Ts/1 -> Product/2
  Gain/1 -> Product/1

== system VtP_mod_3Bit/VCO_3Bit_Quantizer/Discrete-Time VCO2/Compute discrete sample time ==
  In1 : Inport
  Probe : Probe  ProbeWidth=off  ProbeComplexSignal=off
  Submatrix : dspmtrx3/Submatrix  RowSpan=One row  RowStartMode=First  RowStartIndex=1  RowEndMode=Last  RowEndIndex=1  ColSpan=One column  ColStartMode=First  ColStartIndex=1  ColEndMode=Last  ColEndIndex=1
  Out1 : Outport
  wires:
  Submatrix/1 -> Out1/1
  In1/1 -> Probe/1
  Probe/1 -> Submatrix/1

== system VtP_mod_3Bit/VCO_3Bit_Quantizer/Discrete-Time VCO2/Sensitivity ==
  In : Inport
  Ts : Inport  Port=2
  Gain : Gain  Gain=KcRadPerV  ParamDataTypeStr=float('double')  SaturateOnIntegerOverflow=on  OutDataTypeStr=Inherit: Same as input
  Product : Product  RndMeth=Nearest  SaturateOnIntegerOverflow=on  OutDataTypeStr=Inherit: Same as first input
  Out1 : Outport
  wires:
  Product/1 -> Out1/1
  In/1 -> Gain/1
  Ts/1 -> Product/2
  Gain/1 -> Product/1

== system VtP_mod_3Bit/VCO_3Bit_Quantizer/Discrete-Time VCO3/Compute discrete sample time ==
  In1 : Inport
  Probe : Probe  ProbeWidth=off  ProbeComplexSignal=off
  Submatrix : dspmtrx3/Submatrix  RowSpan=One row  RowStartMode=First  RowStartIndex=1  RowEndMode=Last  RowEndIndex=1  ColSpan=One column  ColStartMode=First  ColStartIndex=1  ColEndMode=Last  ColEndIndex=1
  Out1 : Outport
  wires:
  Submatrix/1 -> Out1/1
  In1/1 -> Probe/1
  Probe/1 -> Submatrix/1

== system VtP_mod_3Bit/VCO_3Bit_Quantizer/Discrete-Time VCO3/Sensitivity ==
  In : Inport
  Ts : Inport  Port=2
  Gain : Gain  Gain=KcRadPerV  ParamDataTypeStr=float('double')  SaturateOnIntegerOverflow=on  OutDataTypeStr=Inherit: Same as input
  Product : Product  RndMeth=Nearest  SaturateOnIntegerOverflow=on  OutDataTypeStr=Inherit: Same as first input
  Out1 : Outport
  wires:
  Product/1 -> Out1/1
  In/1 -> Gain/1
  Ts/1 -> Product/2
  Gain/1 -> Product/1

== system VtP_mod_3Bit/VCO_3Bit_Quantizer/Discrete-Time VCO4/Compute discrete sample time ==
  In1 : Inport
  Probe : Probe  ProbeWidth=off  ProbeComplexSignal=off
  Submatrix : dspmtrx3/Submatrix  RowSpan=One row  RowStartMode=First  RowStartIndex=1  RowEndMode=Last  RowEndIndex=1  ColSpan=One column  ColStartMode=First  ColStartIndex=1  ColEndMode=Last  ColEndIndex=1
  Out1 : Outport
  wires:
  Submatrix/1 -> Out1/1
  In1/1 -> Probe/1
  Probe/1 -> Submatrix/1

== system VtP_mod_3Bit/VCO_3Bit_Quantizer/Discrete-Time VCO4/Sensitivity ==
  In : Inport
  Ts : Inport  Port=2
  Gain : Gain  Gain=KcRadPerV  ParamDataTypeStr=float('double')  SaturateOnIntegerOverflow=on  OutDataTypeStr=Inherit: Same as input
  Product : Product  RndMeth=Nearest  SaturateOnIntegerOverflow=on  OutDataTypeStr=Inherit: Same as first input
  Out1 : Outport
  wires:
  Product/1 -> Out1/1
  In/1 -> Gain/1
  Ts/1 -> Product/2
  Gain/1 -> Product/1

== system VtP_mod_3Bit/VCO_3Bit_Quantizer/Discrete-Time VCO5/Compute discrete sample time ==
  In1 : Inport
  Probe : Probe  ProbeWidth=off  ProbeComplexSignal=off
  Submatrix : dspmtrx3/Submatrix  RowSpan=One row  RowStartMode=First  RowStartIndex=1  RowEndMode=Last  RowEndIndex=1  ColSpan=One column  ColStartMode=First  ColStartIndex=1  ColEndMode=Last  ColEndIndex=1
  Out1 : Outport
  wires:
  Submatrix/1 -> Out1/1
  In1/1 -> Probe/1
  Probe/1 -> Submatrix/1

== system VtP_mod_3Bit/VCO_3Bit_Quantizer/Discrete-Time VCO5/Sensitivity ==
  In : Inport
  Ts : Inport  Port=2
  Gain : Gain  Gain=KcRadPerV  ParamDataTypeStr=float('double')  SaturateOnIntegerOverflow=on  OutDataTypeStr=Inherit: Same as input
  Product : Product  RndMeth=Nearest  SaturateOnIntegerOverflow=on  OutDataTypeStr=Inherit: Same as first input
  Out1 : Outport
  wires:
  Product/1 -> Out1/1
  In/1 -> Gain/1
  Ts/1 -> Product/2
  Gain/1 -> Product/1

== system VtP_mod_3Bit/VCO_3Bit_Quantizer/Discrete-Time VCO6/Compute discrete sample time ==
  In1 : Inport
  Probe : Probe  ProbeWidth=off  ProbeComplexSignal=off
  Submatrix : dspmtrx3/Submatrix  RowSpan=One row  RowStartMode=First  RowStartIndex=1  RowEndMode=Last  RowEndIndex=1  ColSpan=One column  ColStartMode=First  ColStartIndex=1  ColEndMode=Last  ColEndIndex=1
  Out1 : Outport
  wires:
  Submatrix/1 -> Out1/1
  In1/1 -> Probe/1
  Probe/1 -> Submatrix/1

== system VtP_mod_3Bit/VCO_3Bit_Quantizer/Discrete-Time VCO6/Sensitivity ==
  In : Inport
  Ts : Inport  Port=2
  Gain : Gain  Gain=KcRadPerV  ParamDataTypeStr=float('double')  SaturateOnIntegerOverflow=on  OutDataTypeStr=Inherit: Same as input
  Product : Product  RndMeth=Nearest  SaturateOnIntegerOverflow=on  OutDataTypeStr=Inherit: Same as first input
  Out1 : Outport
  wires:
  Product/1 -> Out1/1
  In/1 -> Gain/1
  Ts/1 -> Product/2
  Gain/1 -> Product/1

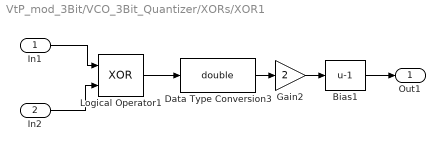
== system VtP_mod_3Bit/VCO_3Bit_Quantizer/XORs/XOR1 ==
  In1 : Inport
  In2 : Inport  Port=2
  Bias1 : Bias  Bias=-1
  Data Type Conversion3 : DataTypeConversion  OutDataTypeStr=double  SampleTime=1/Fs
  Gain2 : Gain  Gain=2  SampleTime=1/Fs
  Logical Operator1 : Logic  Operator=XOR  IconShape=distinctive  AllPortsSameDT=off  OutDataTypeStr=boolean  SampleTime=1/Fs
  Out1 : Outport
  wires:
  Logical Operator1/1 -> Data Type Conversion3/1
  Data Type Conversion3/1 -> Gain2/1
  Gain2/1 -> Bias1/1
  Bias1/1 -> Out1/1
  In2/1 -> Logical Operator1/2
  In1/1 -> Logical Operator1/1

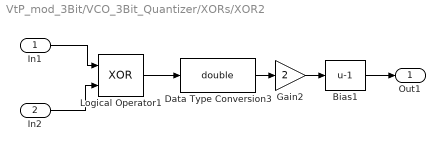
== system VtP_mod_3Bit/VCO_3Bit_Quantizer/XORs/XOR2 ==
  In1 : Inport
  In2 : Inport  Port=2
  Bias1 : Bias  Bias=-1
  Data Type Conversion3 : DataTypeConversion  OutDataTypeStr=double  SampleTime=1/Fs
  Gain2 : Gain  Gain=2  SampleTime=1/Fs
  Logical Operator1 : Logic  Operator=XOR  IconShape=distinctive  AllPortsSameDT=off  OutDataTypeStr=boolean  SampleTime=1/Fs
  Out1 : Outport
  wires:
  Logical Operator1/1 -> Data Type Conversion3/1
  Data Type Conversion3/1 -> Gain2/1
  Gain2/1 -> Bias1/1
  Bias1/1 -> Out1/1
  In2/1 -> Logical Operator1/2
  In1/1 -> Logical Operator1/1

== system VtP_mod_3Bit/VCO_3Bit_Quantizer/XORs/XOR3 ==
  In1 : Inport
  In2 : Inport  Port=2
  Bias1 : Bias  Bias=-1
  Data Type Conversion3 : DataTypeConversion  OutDataTypeStr=double  SampleTime=1/Fs
  Gain2 : Gain  Gain=2  SampleTime=1/Fs
  Logical Operator1 : Logic  Operator=XOR  IconShape=distinctive  AllPortsSameDT=off  OutDataTypeStr=boolean  SampleTime=1/Fs
  Out1 : Outport
  wires:
  Logical Operator1/1 -> Data Type Conversion3/1
  Data Type Conversion3/1 -> Gain2/1
  Gain2/1 -> Bias1/1
  Bias1/1 -> Out1/1
  In2/1 -> Logical Operator1/2
  In1/1 -> Logical Operator1/1

== system VtP_mod_3Bit/VCO_3Bit_Quantizer/XORs/XOR4 ==
  In1 : Inport
  In2 : Inport  Port=2
  Bias1 : Bias  Bias=-1
  Data Type Conversion3 : DataTypeConversion  OutDataTypeStr=double  SampleTime=1/Fs
  Gain2 : Gain  Gain=2  SampleTime=1/Fs
  Logical Operator1 : Logic  Operator=XOR  IconShape=distinctive  AllPortsSameDT=off  OutDataTypeStr=boolean  SampleTime=1/Fs
  Out1 : Outport
  wires:
  Logical Operator1/1 -> Data Type Conversion3/1
  Data Type Conversion3/1 -> Gain2/1
  Gain2/1 -> Bias1/1
  Bias1/1 -> Out1/1
  In2/1 -> Logical Operator1/2
  In1/1 -> Logical Operator1/1

== system VtP_mod_3Bit/VCO_3Bit_Quantizer/XORs/XOR5 ==
  In1 : Inport
  In2 : Inport  Port=2
  Bias1 : Bias  Bias=-1
  Data Type Conversion3 : DataTypeConversion  OutDataTypeStr=double  SampleTime=1/Fs
  Gain2 : Gain  Gain=2  SampleTime=1/Fs
  Logical Operator1 : Logic  Operator=XOR  IconShape=distinctive  AllPortsSameDT=off  OutDataTypeStr=boolean  SampleTime=1/Fs
  Out1 : Outport
  wires:
  Logical Operator1/1 -> Data Type Conversion3/1
  Data Type Conversion3/1 -> Gain2/1
  Gain2/1 -> Bias1/1
  Bias1/1 -> Out1/1
  In2/1 -> Logical Operator1/2
  In1/1 -> Logical Operator1/1

== system VtP_mod_3Bit/VCO_3Bit_Quantizer/XORs/XOR6 ==
  In1 : Inport
  In2 : Inport  Port=2
  Bias1 : Bias  Bias=-1
  Data Type Conversion3 : DataTypeConversion  OutDataTypeStr=double  SampleTime=1/Fs
  Gain2 : Gain  Gain=2  SampleTime=1/Fs
  Logical Operator1 : Logic  Operator=XOR  IconShape=distinctive  AllPortsSameDT=off  OutDataTypeStr=boolean  SampleTime=1/Fs
  Out1 : Outport
  wires:
  Logical Operator1/1 -> Data Type Conversion3/1
  Data Type Conversion3/1 -> Gain2/1
  Gain2/1 -> Bias1/1
  Bias1/1 -> Out1/1
  In2/1 -> Logical Operator1/2
  In1/1 -> Logical Operator1/1

== system VtP_mod_3Bit/VCO_3Bit_Quantizer/XORs/XOR8 ==
  In1 : Inport
  In2 : Inport  Port=2
  Bias1 : Bias  Bias=-1
  Data Type Conversion3 : DataTypeConversion  OutDataTypeStr=double  SampleTime=1/Fs
  Gain2 : Gain  Gain=2  SampleTime=1/Fs
  Logical Operator1 : Logic  Operator=XOR  IconShape=distinctive  AllPortsSameDT=off  OutDataTypeStr=boolean  SampleTime=1/Fs
  Out1 : Outport
  wires:
  Logical Operator1/1 -> Data Type Conversion3/1
  Data Type Conversion3/1 -> Gain2/1
  Gain2/1 -> Bias1/1
  Bias1/1 -> Out1/1
  In2/1 -> Logical Operator1/2
  In1/1 -> Logical Operator1/1
